simulink model "gm_sampleModel1468_sub_sub_sub"  (R2023a)
settings: Solver=VariableStepAuto  StartTime=0.0  StopTime=10.0  RelTol=1e-3
libraries: hdlsllib x4, simulink x2
settings Model: Creator=user1  LastModifiedBy=user1
settings OptimizationCC: BlockReduction=off  ConditionallyExecuteInputs=off
settings DebuggingCC: InheritedTsInSrcMsg=none

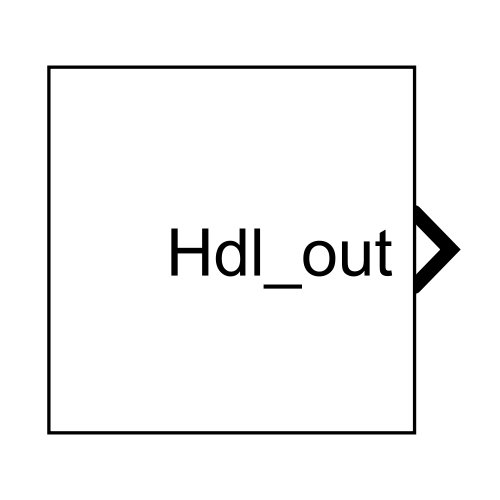
[thumbnail: Simulink's stored preview of the top-level diagram]
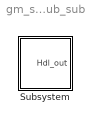
== system gm_sampleModel1468_sub_sub_sub ==
  Subsystem : Subsystem

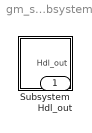
== system gm_sampleModel1468_sub_sub_sub/Subsystem ==
  Subsystem : Subsystem
  Hdl_out : Outport  OutDataTypeStr=uint8

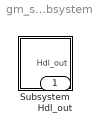
== system gm_sampleModel1468_sub_sub_sub/Subsystem/Subsystem ==
  Subsystem : Subsystem
  Hdl_out : Outport  OutDataTypeStr=uint8

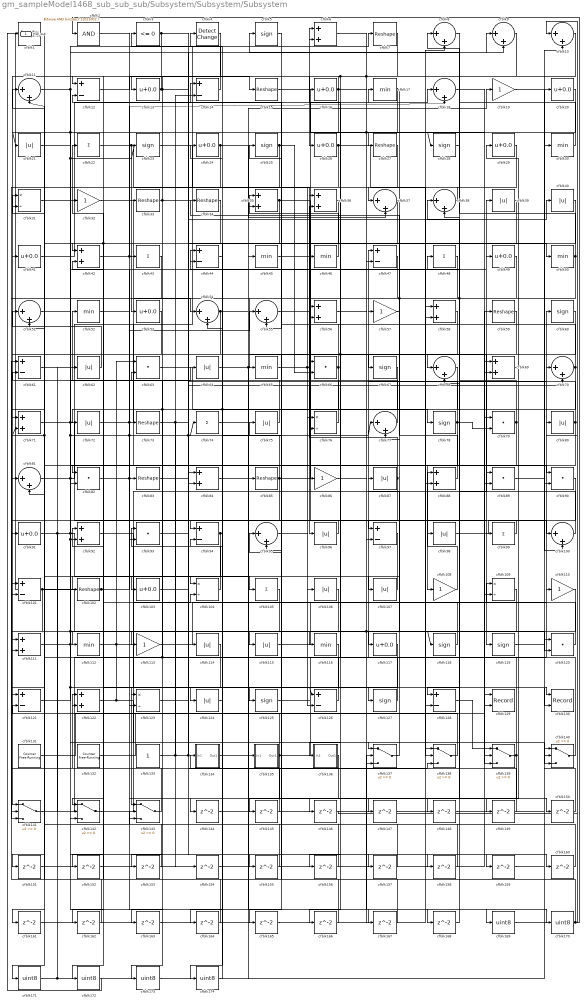
== system gm_sampleModel1468_sub_sub_sub/Subsystem/Subsystem/Subsystem ==
  cfblk1 : hdlsllib/Logic and Bit Operations/Detect Rise Nonnegative  vinit=0  OutDataTypeStr=uint8
  cfblk{8..11,18,37..38,51,54..55,68,70,77,81,95,100} (16 alike) : Sum  Inputs=|++  OutDataTypeStr=uint8
  cfblk{12,14,44,47,61,94,97,101,121,126,128} (11 alike) : Sum  Inputs=+-  OutDataTypeStr=uint8
  cfblk{7,15,27,33..34,59,73,83,85,102} (10 alike) : Reshape
  cfblk{13,16,20,24,26,29,41,49,53,91,103,117} (12 alike) : Bias  Bias=0.0  SaturateOnIntegerOverflow=off
  cfblk{31,76,104,109,123} (5 alike) : Product  Inputs=*/  OutDataTypeStr=uint8  RndMeth=Zero  SaturateOnIntegerOverflow=on
  cfblk{22,43,48,74,99,105} (6 alike) : Sum  Inputs=+  OutDataTypeStr=uint8
  cfblk{21,39..40,62,64,72,75,80,87,96,98,106..107,114..115,124} (16 alike) : Abs  OutDataTypeStr=uint8  SaturateOnIntegerOverflow=off
  cfblk{19,32,57,86,108,110,113} (7 alike) : Gain  OutDataTypeStr=uint8
  cfblk{6,35..36,42,56,58,69,71,84,88,92,111,122} (13 alike) : Sum  OutDataTypeStr=uint8
  cfblk{17,30,45..46,50,52,65,112,116} (9 alike) : MinMax  OutDataTypeStr=uint8
  cfblk{5,23,25,28,60,67,78,118..119,125,127} (11 alike) : Signum
  cfblk{63,66,79,82,89..90,93,120} (8 alike) : DotProduct  OutDataTypeStr=uint8
  cfblk129 : Record  FileSettingsInternal="{\"entries\":[{\"content\":{\"excelSettings\":{\"content\":{},\"type\":\"Streamout.ExcelSettings\"}},\"type\":\"Streamout.FileSettingStorage\",\"uuid\":\"\"}],\"packageUris\":[\"http:\\/\\/schema.mathworks.com\\/mf0\\/streamout_blocks\\/R2020a\"],\"version\":\"1.0\"}"  Layout=[1 1]  SignalsInternal="{\"entries\":[{\"content\":{\"signals\":[{\"content\":{\"blockPath\":[],\"dimensions\":[1],\"domain\":\"\",\"lineColor\":\"#a2142f\",\"plots\":[1],\"port\":1,\"signalID\":19746,\"signalName\":\"cfblk18\"},\"type\":\"RecordBlkView.Signal\",\"uuid\":\"\"},{\"content\":{\"blockPath\":[],\"dimensions\":[1],\"domain\":\"\",\"lineColor\":\"#139fff\",\"plots\":[1],\"port\":2,\"signalID\":19749,\"signalName\":\"cfblk65\"},\"type\":\"RecordBlkView.Signal\",\"uuid\":\"\"}]},\"type\":\"RecordBlkView.InputSignals\",\"uuid\":\"\"}],\"packageUris\":[\"http:\\/\\/schema.mathworks.com\\/mf0\\/streamout_blocks\\/R2020a\"],\"version\":\"1.0\"}"  VisualizationBindings="{\"xyplotplugin\":{\"info\":[{\"series\":[{\"bindingParametersList\":[{\"parameter\":\"X-Axis\",\"signalID\":19746,\"signalName\":\"cfblk18\"},{\"parameter\":\"Y-Axis\",\"signalID\":19749,\"signalName\":\"cfblk65\"}],\"seriesID\":43273}],\"subplotID\":1}]}}"  CompatibilityTag=XY  st=-1
  cfblk130 : Record  FileSettingsInternal="{\"entries\":[{\"content\":{\"excelSettings\":{\"content\":{},\"type\":\"Streamout.ExcelSettings\"}},\"type\":\"Streamout.FileSettingStorage\",\"uuid\":\"\"}],\"packageUris\":[\"http:\\/\\/schema.mathworks.com\\/mf0\\/streamout_blocks\\/R2020a\"],\"version\":\"1.0\"}"  Layout=[1 1]  SignalsInternal="{\"entries\":[{\"content\":{\"signals\":[{\"content\":{\"blockPath\":[],\"dimensions\":[1],\"domain\":\"\",\"lineColor\":\"#a2142f\",\"plots\":[1],\"port\":1,\"signalID\":19754,\"signalName\":\"cfblk92\"},\"type\":\"RecordBlkView.Signal\",\"uuid\":\"\"},{\"content\":{\"blockPath\":[],\"dimensions\":[1],\"domain\":\"\",\"lineColor\":\"#139fff\",\"plots\":[1],\"port\":2,\"signalID\":19757,\"signalName\":\"cfblk73\"},\"type\":\"RecordBlkView.Signal\",\"uuid\":\"\"}]},\"type\":\"RecordBlkView.InputSignals\",\"uuid\":\"\"}],\"packageUris\":[\"http:\\/\\/schema.mathworks.com\\/mf0\\/streamout_blocks\\/R2020a\"],\"version\":\"1.0\"}"  VisualizationBindings="{\"xyplotplugin\":{\"info\":[{\"series\":[{\"bindingParametersList\":[{\"parameter\":\"X-Axis\",\"signalID\":19754,\"signalName\":\"cfblk92\"},{\"parameter\":\"Y-Axis\",\"signalID\":19757,\"signalName\":\"cfblk73\"}],\"seriesID\":41793}],\"subplotID\":1}]}}"  CompatibilityTag=XY  st=-1
  cfblk131 : hdlsllib/Sources/Counter Free-Running  NumBits=16  tsamp=-1
  cfblk132 : hdlsllib/Sources/Counter Free-Running  NumBits=16  tsamp=-1
  cfblk133 : Constant  OutDataTypeStr=uint8  SampleTime=-1
  cfblk134 : Subsystem
      settings: LibrarySourceBlock=|
      | hdlsllib/Ports &
      | Subsystems/Subsystem
  cfblk135 : Subsystem
      settings: LibrarySourceBlock=|
      | hdlsllib/Ports &
      | Subsystems/Subsystem
  cfblk136 : Subsystem
      settings: LibrarySourceBlock=|
      | hdlsllib/Ports &
      | Subsystems/Subsystem
  cfblk{137..143} (7 alike) : Switch  OutDataTypeStr=uint8  SaturateOnIntegerOverflow=off  InputSameDT=off
  cfblk{144..168} (25 alike) : Delay  SampleTime=1
  cfblk{169..174} (6 alike) : DataTypeConversion  OutDataTypeStr=uint8  SaturateOnIntegerOverflow=off  RndMeth=Floor
  cfblk2 : simulink/Logic and Bit Operations/Bitwise Operator  logicop=AND  UseBitMask=on  BitMask=bin2dec('11011001')  BitMaskRealWorld=Stored Integer
      settings: LibrarySourceBlock=|
      | hdlsllib/Logic and Bit
      | Operations/Bitwise
      | Operator
  cfblk3 : hdlsllib/Logic and Bit Operations/Compare To Zero  relop=<=  OutDataTypeStr=uint8
  cfblk4 : simulink/Logic and Bit Operations/Detect Change  vinit=0  OutDataTypeStr=uint8
      settings: LibrarySourceBlock=|
      | hdlsllib/Logic and Bit
      | Operations/Detect
      | Change
  Hdl_out : Outport  OutDataTypeStr=uint8
  wires:
  cfblk174/1 -> cfblk4/1
  cfblk173/1 -> cfblk20/1
  cfblk4/1 -> cfblk173/1
  cfblk172/1 -> cfblk1/1
  cfblk114/1 -> cfblk172/1
  cfblk171/1 -> cfblk85/1, cfblk62/1
  cfblk170/1 -> cfblk80/1, cfblk134/1(In1)
  cfblk169/1 -> cfblk2/1
  cfblk168/1 -> cfblk38/1
  cfblk167/1 -> cfblk95/1
  cfblk21/1 -> cfblk167/1
  cfblk166/1 -> cfblk122/2
  cfblk165/1 -> cfblk58/1
  cfblk136/1(Out1) -> cfblk165/1
  cfblk164/1 -> cfblk101/1
  cfblk117/1 -> cfblk164/1
  cfblk163/1 -> cfblk137/3
  cfblk162/1 -> cfblk31/2
  cfblk161/1 -> cfblk8/2
  cfblk160/1 -> cfblk121/2
  cfblk159/1 -> cfblk120/1
  cfblk83/1 -> cfblk159/1
  cfblk158/1 -> cfblk137/2
  cfblk157/1 -> cfblk35/2
  cfblk156/1 -> cfblk11/1
  cfblk155/1 -> cfblk143/2
  cfblk154/1 -> cfblk54/2
  cfblk153/1 -> cfblk42/2
  cfblk109/1 -> cfblk153/1
  cfblk152/1 -> cfblk89/2
  cfblk53/1 -> cfblk152/1
  cfblk151/1 -> cfblk88/2
  cfblk150/1 -> cfblk140/1
  cfblk56/1 -> cfblk150/1
  cfblk149/1 -> cfblk61/1
  cfblk148/1 -> cfblk69/1
  cfblk110/1 -> cfblk148/1
  cfblk147/1 -> cfblk138/1
  cfblk84/1 -> cfblk147/1
  cfblk146/1 -> cfblk10/1
  cfblk145/1 -> cfblk51/2
  cfblk68/1 -> cfblk145/1
  cfblk144/1 -> cfblk140/2
  cfblk124/1 -> cfblk144/1
  cfblk44/1 -> cfblk24/1
  cfblk49/1 -> cfblk117/1, cfblk136/1(In1), cfblk128/1
  cfblk9/1 -> cfblk102/1
  cfblk67/1 -> cfblk86/1
  cfblk46/1 -> cfblk35/1
  cfblk106/1 -> cfblk116/1
  cfblk58/1 -> cfblk82/1, cfblk166/1
  cfblk143/1 -> cfblk122/1
  cfblk38/1 -> cfblk33/1
  cfblk34/1 -> cfblk142/1, cfblk111/1
  cfblk94/1 -> cfblk44/2, cfblk151/1
  cfblk17/1 -> cfblk27/1, cfblk77/2
  cfblk75/1 -> cfblk31/1
  cfblk5/1 -> cfblk55/2
  cfblk120/1 -> cfblk32/1
  cfblk111/1 -> cfblk9/2, cfblk23/1, cfblk128/2
  cfblk127/1 -> cfblk16/1
  cfblk43/1 -> cfblk101/2
  cfblk102/1 -> cfblk55/1, Hdl_out/1
  cfblk133/1 -> cfblk138/3, cfblk70/2, cfblk14/2
  cfblk26/1 -> cfblk138/2, cfblk142/3
  cfblk57/1 -> cfblk107/1
  cfblk119/1 -> cfblk30/1
  cfblk61/1 -> cfblk120/2, cfblk160/1
  cfblk18/1 -> cfblk129/1
  cfblk104/1 -> cfblk93/1
  cfblk87/1 -> cfblk36/2, cfblk121/1
  cfblk74/1 -> cfblk139/3
  cfblk24/1 -> cfblk37/2, cfblk72/1
  cfblk60/1 -> cfblk95/2
  cfblk59/1 -> cfblk115/1
  cfblk65/1 -> cfblk67/1, cfblk129/2
  cfblk138/1 -> cfblk61/2
  cfblk118/1 -> cfblk94/2
  cfblk14/1 -> cfblk3/1
  cfblk45/1 -> cfblk69/2
  cfblk12/1 -> cfblk15/1
  cfblk93/1 -> cfblk40/1, cfblk77/1
  cfblk90/1 -> cfblk109/2
  cfblk137/1 -> cfblk87/1
  cfblk55/1 -> cfblk139/2
  cfblk131/1 -> cfblk114/1
  cfblk31/1 -> cfblk22/1
  cfblk28/1 -> cfblk68/2
  cfblk89/1 -> cfblk10/2
  cfblk80/1 -> cfblk56/1, cfblk149/1
  cfblk122/1 -> cfblk137/1, cfblk63/1
  cfblk52/1 -> cfblk73/1, cfblk155/1
  cfblk51/1 -> cfblk140/3, cfblk126/1
  cfblk95/1 -> cfblk106/1
  cfblk40/1 -> cfblk47/2
  cfblk113/1 -> cfblk45/1
  cfblk140/1 -> cfblk75/1
  cfblk103/1 -> cfblk70/1
  cfblk39/1 -> cfblk42/1
  cfblk88/1 -> cfblk34/1
  cfblk115/1 -> cfblk109/1
  cfblk2/1 -> cfblk170/1
  cfblk107/1 -> cfblk103/1
  cfblk16/1 -> cfblk21/1, cfblk82/2, cfblk28/1, cfblk99/1, cfblk13/1
  cfblk50/1 -> cfblk5/1, cfblk58/2
  cfblk82/1 -> cfblk49/1, cfblk74/1, cfblk98/1
  cfblk7/1 -> cfblk84/2, cfblk156/1, cfblk97/2
  cfblk1/1 -> cfblk171/1
  cfblk8/1 -> cfblk38/2
  cfblk70/1 -> cfblk123/1, cfblk162/1, cfblk174/1, cfblk12/2
  cfblk19/1 -> cfblk100/2
  cfblk36/1 -> cfblk124/1
  cfblk6/1 -> cfblk68/1
  cfblk116/1 -> cfblk143/1
  cfblk11/1 -> cfblk7/1, cfblk90/1
  cfblk71/1 -> cfblk97/1, cfblk157/1
  cfblk25/1 -> cfblk141/3, cfblk66/2
  cfblk69/1 -> cfblk89/1, cfblk29/1
  cfblk105/1 -> cfblk141/2
  cfblk20/1 -> cfblk41/1
  cfblk76/1 -> cfblk25/1
  cfblk15/1 -> cfblk79/1
  cfblk141/1 -> cfblk57/1
  cfblk121/1 -> cfblk92/2, cfblk46/1
  cfblk108/1 -> cfblk88/1
  cfblk126/1 -> cfblk92/1, cfblk63/2
  cfblk47/1 -> cfblk65/1
  cfblk96/1 -> cfblk91/1
  cfblk81/1 -> cfblk9/1, cfblk158/1
  cfblk79/1 -> cfblk44/1, cfblk161/1
  cfblk22/1 -> cfblk43/1, cfblk76/1
  cfblk99/1 -> cfblk94/1
  cfblk134/1(Out1) -> cfblk110/1
  cfblk73/1 -> cfblk130/2, cfblk154/1
  cfblk10/1 -> cfblk26/1
  cfblk132/1 -> cfblk59/1
  cfblk98/1 -> cfblk100/1
  cfblk41/1 -> cfblk6/2
  cfblk42/1 -> cfblk54/1, cfblk18/2
  cfblk92/1 -> cfblk130/1
  cfblk72/1 -> cfblk18/1, cfblk90/2
  cfblk123/1 -> cfblk84/1
  cfblk23/1 -> cfblk36/1
  cfblk100/1 -> cfblk48/1
  cfblk78/1 -> cfblk47/1, cfblk93/2, cfblk79/2
  cfblk101/1 -> cfblk135/1(In1), cfblk111/2
  cfblk125/1 -> cfblk127/1
  cfblk37/1 -> cfblk53/1
  cfblk97/1 -> cfblk104/1
  cfblk32/1 -> cfblk108/1
  cfblk54/1 -> cfblk81/1, cfblk19/1
  cfblk62/1 -> cfblk51/1
  cfblk13/1 -> cfblk50/1, cfblk163/1, cfblk12/1
  cfblk66/1 -> cfblk125/1, cfblk56/2
  cfblk48/1 -> cfblk112/1
  cfblk33/1 -> cfblk6/1, cfblk113/1
  cfblk142/1 -> cfblk39/1
  cfblk91/1 -> cfblk76/2, cfblk64/1, cfblk105/1, cfblk142/2
  cfblk63/1 -> cfblk78/1
  cfblk29/1 -> cfblk96/1
  cfblk139/1 -> cfblk11/2, cfblk71/2, cfblk146/1
  cfblk112/1 -> cfblk83/1, cfblk104/2
  cfblk86/1 -> cfblk118/1, cfblk169/1
  cfblk128/1 -> cfblk139/1
  cfblk3/1 -> cfblk141/1, cfblk126/2
  cfblk64/1 -> cfblk66/1, cfblk168/1
  cfblk85/1 -> cfblk17/1, cfblk14/1, cfblk123/2
  cfblk135/1(Out1) -> cfblk60/1, cfblk81/2, cfblk143/3
  cfblk35/1 -> cfblk119/1, cfblk71/1
  cfblk30/1 -> cfblk8/1
  cfblk77/1 -> cfblk52/1
  cfblk27/1 -> cfblk37/1

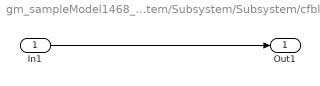
== system gm_sampleModel1468_sub_sub_sub/Subsystem/Subsystem/Subsystem/cfblk134 ==
  In1 : Inport
  Out1 : Outport
  wires:
  In1/1 -> Out1/1

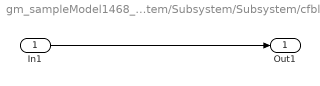
== system gm_sampleModel1468_sub_sub_sub/Subsystem/Subsystem/Subsystem/cfblk135 ==
  In1 : Inport
  Out1 : Outport
  wires:
  In1/1 -> Out1/1

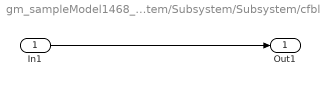
== system gm_sampleModel1468_sub_sub_sub/Subsystem/Subsystem/Subsystem/cfblk136 ==
  In1 : Inport
  Out1 : Outport
  wires:
  In1/1 -> Out1/1
